simulink model "quadcopter_mpc_position_test"  (R2015b)
settings: Solver=VariableStepAuto  StartTime=0.0  StopTime=30  RelTol=1e-3
undefined symbols (not defined in the file): md_quadcopter, seed
libraries: vrlib x2
settings Model: Creator=Daniel  LastModifiedBy=Daniel
settings SolverCC: AlgebraicLoopSolver=LineSearch

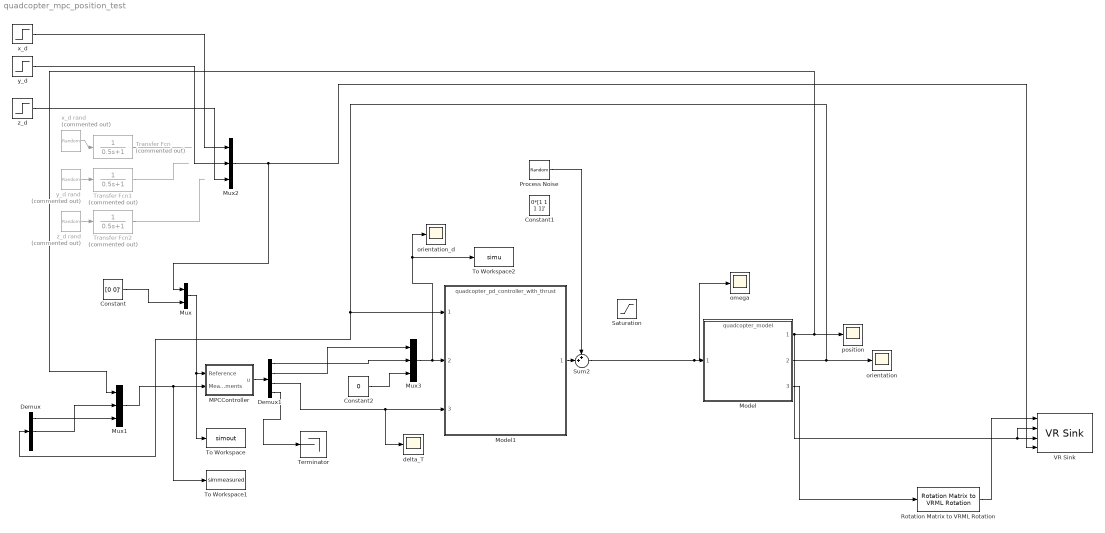
== system quadcopter_mpc_position_test ==
  Constant : Constant  Value=[0 0]'
  Constant1 : Constant  Value=0*[1 1 1 1]'
  Constant2 : Constant  Value=0
  Demux : Demux  Outputs=3
  Demux1 : Demux
  MPCController : Subsystem  mask{md=md_quadcopter}
      mask prompts: md "MPCData"
  Model : ModelReference  ModelNameDialog=quadcopter_model.mdl  SimulationMode=Normal  ModelReferenceVersion=1.113  CopyOfModelName=quadcopter_model.mdl
  Model1 : ModelReference  ModelNameDialog=quadcopter_pd_controller_with_thrust.mdl  SimulationMode=Normal  ModelReferenceVersion=1.70  CopyOfModelName=quadcopter_pd_controller_with_thrust.mdl
  Mux : Mux  Inputs=2
  Mux1 : Mux  Inputs=3
  Mux2 : Mux  Inputs=3
  Mux3 : Mux  Inputs=3
  Process Noise : RandomNumber  Mean=[0 0 0 0]'  Variance=0
  Rotation Matrix to VRML Rotation : vrlib/Utilities/Rotation Matrix to VRML Rotation  maxzero=1e-12
  Saturation : Saturate  UpperLimit=900  LowerLimit=0
  Sum2 : Sum  Inputs=++|
  Terminator : Terminator
  To Workspace : ToWorkspace  VariableName=simout  SaveFormat=Timeseries  SampleTime=-1
  To Workspace1 : ToWorkspace  VariableName=simmeasured  SaveFormat=Timeseries  SampleTime=-1
  To Workspace2 : ToWorkspace  VariableName=simu  SaveFormat=Timeseries  SampleTime=-1
  Transfer Fcn : TransferFcn  Commented=on  Denominator=[0.5 1]
  Transfer Fcn1 : TransferFcn  Commented=on  Denominator=[0.5 1]
  Transfer Fcn2 : TransferFcn  Commented=on  Denominator=[0.5 1]
  VR Sink : vrlib/VR Sink  InstantiateOnLoad=on  SampleTime=0.05  ViewEnable=on  RemoteChange=off  RemoteView=off  FieldsWritten=copter.rotation.4.1.1.double#copter.translation.3.1.1.double#vp.translation.3.1.1.double#target.translation.3.1.1.double  WorldFileName=copter_world.wrl  WorldDescription=quadcopter_world  AutoView=on  VideoDimensions=[]  AllowVariableSize=off  FigureProperties="{'Position', 'Name', 'Viewpoint', 'CameraBound', 'CameraDirection', 'CameraPosition', 'CameraUpVector', 'ZoomFactor', 'Antialiasing', 'Headlight', 'Lighting', 'NavPanel', 'Sound', 'StatusBar', 'Stereo3D', 'Stereo3DCameraOffset', 'Stereo3DHIT', 'ToolBar', 'Textures', 'Transparency', 'Triad', 'Wireframe', 'NavZones', 'NavMode', 'NavSpeed', 'CaptureFileFormat', 'CaptureFileName', 'Record2DCompressMethod', 'Record2DCompressQuality', 'Record2D', 'Record2DFileName', 'Record2DFPS'; [9.5500000000000000e+02   2.9000000000000000e+02   5.7600000000000000e+02   3.8000000000000000e+02], 'quadcopter_world', 'viewpoint', 'on', [0.0000000000000000e+00   0.0000000000000000e+00  -1.0000000000000000e+00], [0.0000000000000000e+00   0.0000000000000000e+00   0.0000000000000000e+00], [0.0000000000000000e+00   1.0000000000000000e+00   0.0000000000000000e+00], [1.0000000000000000e+00], 'on', 'on', 'on', 'halfbar', 'on', 'on', 'off', [1.0000000149011612e-01], [0.0000000000000000e+00], 'on', 'on', 'on', 'none', 'off', 'off', 'fly', 'normal', 'tif', '%f_anim_%n.tif', 'auto', [7.5000000000000000e+01], 'off', '%f_anim_%n.avi', 'auto'}"
  delta_T : Scope
  "omega " : Scope
  orientation : Scope
  orientation_d : Scope
  position : Scope
  x_d : Step  Time=30  After=5  SampleTime=0
  x_d rand : UniformRandomNumber  Commented=on  Minimum=-30  Maximum=30  Seed=0+seed  SampleTime=10
  y_d : Step  Time=30  Before=2  After=5  SampleTime=0
  y_d rand : UniformRandomNumber  Commented=on  Minimum=-30  Maximum=30  Seed=1+seed  SampleTime=10
  z_d : Step  Time=30  After=0  SampleTime=0
  z_d rand : UniformRandomNumber  Commented=on  Minimum=0  Maximum=15  Seed=2+seed  SampleTime=10
  wires:
  Model/2 -> Model1/1, Demux/1, orientation/1
  Model/1 -> Mux1/1, position/1, VR Sink/2, VR Sink/3
  Model/3 -> Rotation Matrix to VRML Rotation/1
  x_d rand/1 -> Transfer Fcn/1
  y_d rand/1 -> Transfer Fcn1/1
  z_d rand/1 -> Transfer Fcn2/1
  Rotation Matrix to VRML Rotation/1 -> VR Sink/1
  Mux2/1 -> Mux/1, VR Sink/4
  Transfer Fcn/1 -> ?
  Transfer Fcn1/1 -> ?
  Transfer Fcn2/1 -> ?
  Process Noise/1 -> Sum2/1
  Model1/1 -> Sum2/2
  Constant/1 -> Mux/2
  Mux/1 -> To Workspace/1, MPCController/1(Reference)
  Demux/2 -> Mux1/2
  Demux/1 -> Mux1/3
  Mux1/1 -> To Workspace1/1, MPCController/2(Measurements)
  MPCController/1(u) -> Demux1/1
  Demux1/3 -> delta_T/1, Model1/3
  Mux3/1 -> To Workspace2/1, orientation_d/1, Model1/2
  Constant2/1 -> Mux3/3
  Demux1/2 -> Mux3/1
  Demux1/1 -> Mux3/2
  z_d/1 -> Mux2/3
  y_d/1 -> Mux2/2
  x_d/1 -> Mux2/1
  Sum2/1 -> Model/1, "omega "/1
  Demux1/4 -> Terminator/1

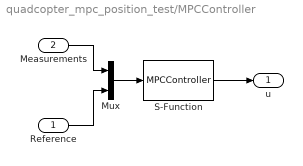
== system quadcopter_mpc_position_test/MPCController ==
  Reference : Inport
  Measurements : Inport  Port=2
  Mux : Mux  Inputs=2
  S-Function : S-Function  FunctionName=MPCController  Parameters=md  SFunctionDeploymentMode=off  EnableBusSupport=off
  u : Outport
  wires:
  S-Function/1 -> u/1
  Reference/1 -> Mux/2
  Measurements/1 -> Mux/1
  Mux/1 -> S-Function/1
